simulink model "ACC_simple_model"  (R2018a)
settings: Solver=FixedStepAuto  StartTime=0.0  StopTime=100  RelTol=1e-3
InitFcn:
  | m       = 1800;     % Total mass of vehicle                          (kg)
  | Iz      = 2875;     % Yaw moment of inertia of vehicle               (m*N*s^2)
  | lf      = 1.2;      % Longitudinal distance from c.g. to front tires (m)
  | lr      = 1.6;      % Longitudinal distance from c.g. to rear tires  (m)
  | Cf      = 19000;    % Cornering stiffness of front tires             (N/rad)
  | Cr      = 33000;    % Cornering stiffness of rear tires              (N/rad)
  | tau     = 0.5;      % Longitudinal time constant                     (N/A)
  | 
  | % Initial condition for the ego car
  | v0_ego = 25.6;         % Initial speed of the ego car           (m/s)
  | x0_ego = 0;            % Initial x position of ego car          (m)
  | y0_ego = -757.8;       % Initial y position of ego car          (m)
libraries: simulink x1
settings Model: Creator=CHIZOM WORNU  LastModifiedBy=CHIZOM WORNU
settings OptimizationCC: DefaultParameterBehavior=Inlined  UseDivisionForNetSlopeComputation=on  UseFloatMulNetSlope=on  InlineInvariantSignals=on  PassReuseOutputArgsAs=Individual arguments  ZeroExternalMemoryAtStartup=off  ZeroInternalMemoryAtStartup=off  NoFixptDivByZeroProtection=on  EfficientFloat2IntCast=on  LifeSpan=1  OptimizeBlockOrder=speed  DifferentSizesBufferReuse=on
settings DebuggingCC: ParameterTunabilityLossMsg=error
settings HardwareCC: ProdLongLongMode=on
settings SFSimCC: MATLABDynamicMemAlloc=off
settings RTWCC: SystemTargetFile=ert.tlc  GenCodeOnly=on  PackageName=Accsimple  TemplateMakefile=ert_default_tmf  GenerateReport=on  Toolchain=Microsoft Visual C++ 2017 v15.0 | nmake (64-bit Windows)  IncludeHyperlinkInReport=on  LaunchReport=on  GenerateTraceInfo=on  GenerateTraceReport=on  GenerateTraceReportSl=on  GenerateTraceReportSf=on  GenerateTraceReportEml=on  GenerateCodeMetricsReport=on
settings CodeAppCC: ForceParamTrailComments=on  IgnoreCustomStorageClasses=off  OperatorAnnotations=on  SimulinkDataObjDesc=on  SFDataObjDesc=on  CustomSymbolStrGlobalVar=rt$N$M  CustomSymbolStrType=$N$M  CustomSymbolStrFcn=$N$M$F  CustomSymbolStrMacro=$N$M  InsertBlockDesc=on
settings ERTTargetCC: TargetLangStandard=C99 (ISO)  GenerateSampleERTMain=on  IncludeMdlTerminateFcn=off  CombineSignalStateStructs=on  SupportComplex=off  SupportContinuousTime=on  InlinedParameterPlacement=NonHierarchical  ERTCustomFileTemplate=example_file_process.tlc

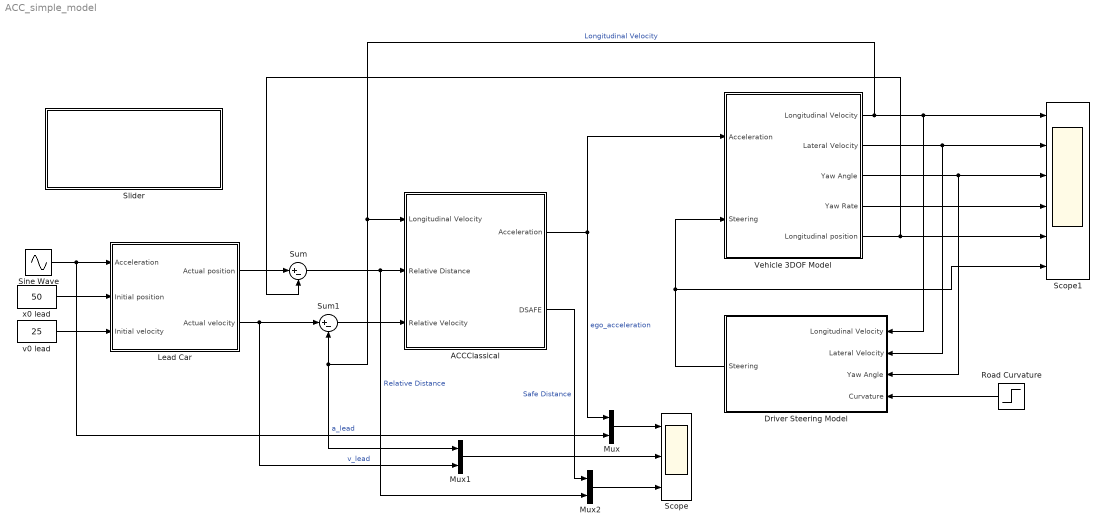
== system ACC_simple_model ==
  "  Vehicle 3DOF Model " : Subsystem
  ACCClassical : Subsystem  TreatAsAtomicUnit=on  VariantControl=controller_type == 1
      settings: RTWFileNameOpts=Use function name
  Driver Steering Model : Subsystem
  Lead Car : Subsystem
  Mux : Mux  Inputs=2
  Mux1 : Mux  Inputs=2
  Mux2 : Mux  Inputs=2
  Road Curvature : Step  Time=50  Before=1/760  After=4/760  SampleTime=0
  Scope : Scope  NumInputPorts=3
  Scope1 : Scope  NumInputPorts=6
  Sine Wave : Sin  Amplitude=0.3188405797101  Frequency=0.2  SampleTime=0.1
  Slider : Subsystem  DialogController=hmiCreateDDGDialog  IsWebBlock=on  mask(MWDashboardBlock){webBlockId=eaa1054b-b6c0-4885-96b6-8836a32feb3e, webBlockType=slider, ShowInLibBrowser=on, ShowInitialText=on, HMISrcModelName=ACC_simple_model}
      mask prompts: webBlockId "WebBlock Id"; webBlockType "WebBlock Type"; HMISrcModelName "Source Model"
      mask help: SimulinkHMI:dialogs:SliderDialogDesc
      mask Help: helpview([docroot '/mapfiles/simulink.map'], 'hmi_slider')
      mask Display:
      | if strcmp(get_param(bdroot(gcb),'BlockDiagramType'), 'library')
      |     image([(matlabroot) '/toolbox/simulink/hmi/icons/Slider.png']);
      | end
  Sum : Sum  Inputs=|+-
  Sum1 : Sum  Inputs=|+-
  v0 lead : Constant  Value=25  SampleTime=0.1
  x0 lead : Constant  Value=50  SampleTime=0.1
  wires:
  Lead Car/2(Actual velocity) -> Sum1/1, Mux1/2  "v_lead"
  Sine Wave/1 -> Mux/2, Lead Car/1(Acceleration)  "a_lead"
  Lead Car/1(Actual position) -> Sum/1
  v0 lead/1 -> Lead Car/3(Initial velocity)
  x0 lead/1 -> Lead Car/2(Initial position)
  ACCClassical/1(Acceleration) -> "  Vehicle 3DOF Model "/1(Acceleration), Mux/1  "ego_acceleration"
  ACCClassical/2("DSAFE ") -> Mux2/1  "Safe Distance"
  Driver Steering Model/1(Steering) -> "  Vehicle 3DOF Model "/2(Steering), Scope1/6
  "  Vehicle 3DOF Model "/1(Longitudinal Velocity) -> Driver Steering Model/1(Longitudinal Velocity), Scope1/1, ACCClassical/1(Longitudinal Velocity), Mux1/1, Sum1/2  "Longitudinal Velocity"
  "  Vehicle 3DOF Model "/2(Lateral Velocity) -> Driver Steering Model/2(Lateral Velocity), Scope1/2
  "  Vehicle 3DOF Model "/3(Yaw Angle) -> Driver Steering Model/3(Yaw Angle), Scope1/3
  "  Vehicle 3DOF Model "/4(Yaw Rate) -> Scope1/4
  "  Vehicle 3DOF Model "/5(Longitudinal position) -> Sum/2, Scope1/5
  Road Curvature/1 -> Driver Steering Model/4(Curvature)
  Mux/1 -> Scope/1
  Mux1/1 -> Scope/2
  Mux2/1 -> Scope/3
  Sum1/1 -> ACCClassical/3(Relative Velocity)
  Sum/1 -> ACCClassical/2(Relative Distance), Mux2/2  "Relative Distance"

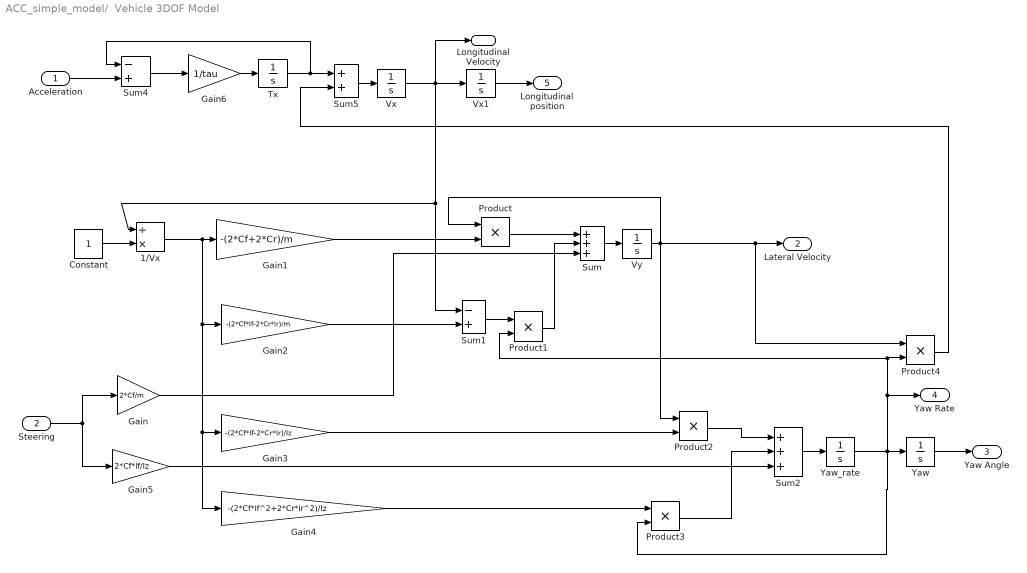
== system ACC_simple_model/  Vehicle 3DOF Model  ==
  Acceleration : Inport
  Steering : Inport  Port=2
  1/Vx : Product  Inputs=/*
  Constant : Constant
  Gain : Gain  Gain=2*Cf/m
  Gain1 : Gain  Gain=-(2*Cf+2*Cr)/m
  Gain2 : Gain  Gain=-(2*Cf*lf-2*Cr*lr)/m
  Gain3 : Gain  Gain=-(2*Cf*lf-2*Cr*lr)/Iz
  Gain4 : Gain  Gain=-(2*Cf*lf^2+2*Cr*lr^2)/Iz
  Gain5 : Gain  Gain=2*Cf*lf/Iz
  Gain6 : Gain  Gain=1/tau
  Product{,1..4} (5 alike) : Product
  Sum : Sum  Inputs=+++
  Sum1 : Sum  Inputs=-+
  Sum2 : Sum  Inputs=+++
  Sum4 : Sum  Inputs=-+
  Sum5 : Sum
  Tx : Integrator
  Vx : Integrator  InitialCondition=v0_ego
  Vx1 : Integrator  InitialCondition=v0_ego
  Vy : Integrator
  Yaw : Integrator
  "Yaw_rate " : Integrator
  Longitudinal Velocity : Outport
  Lateral Velocity : Outport  Port=2
  Yaw Angle : Outport  Port=3
  Yaw Rate : Outport  Port=4
  Longitudinal position : Outport  Port=5
  wires:
  Vx/1 -> 1/Vx/1, Sum1/1, Vx1/1, Longitudinal Velocity/1
  Vy/1 -> Product/1, Product4/1, Lateral Velocity/1, Product2/1
  Yaw/1 -> Yaw Angle/1
  "Yaw_rate "/1 -> Product4/2, Product1/2, Yaw Rate/1, Product3/2, Yaw/1
  Vx1/1 -> Longitudinal position/1
  Product1/1 -> Sum/2
  Sum/1 -> Vy/1
  Product/1 -> Sum/1
  Gain1/1 -> Product/2
  Steering/1 -> Gain/1, Gain5/1
  Gain/1 -> Sum/3
  Sum1/1 -> Product1/1
  Product4/1 -> Sum5/2
  Gain5/1 -> Sum2/3
  Product3/1 -> Sum2/2
  Tx/1 -> Sum5/1, Sum4/1
  Acceleration/1 -> Sum4/2
  Sum4/1 -> Gain6/1
  Product2/1 -> Sum2/1
  1/Vx/1 -> Gain1/1, Gain4/1, Gain3/1, Gain2/1
  Gain3/1 -> Product2/2
  Constant/1 -> 1/Vx/2
  Gain4/1 -> Product3/1
  Gain2/1 -> Sum1/2
  Sum5/1 -> Vx/1
  Sum2/1 -> "Yaw_rate "/1
  Gain6/1 -> Tx/1

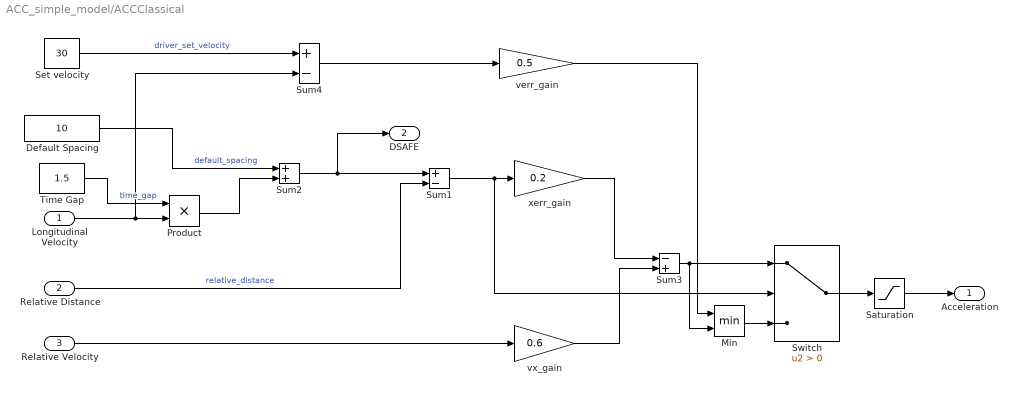
== system ACC_simple_model/ACCClassical ==
  Longitudinal Velocity : Inport
  Relative Distance : Inport  Port=2
  Relative Velocity : Inport  Port=3
  Default Spacing : Constant  Value=10  SampleTime=0.1
  Min : MinMax  Inputs=2
  Product : Product
  Saturation : Saturate  UpperLimit=2  LowerLimit=-3
  Set velocity : Constant  Value=30  SampleTime=0.1
  Sum1 : Sum  Inputs=+-
  Sum2 : Sum
  Sum3 : Sum  Inputs=-+
  Sum4 : Sum  Inputs=+-
  Switch : Switch  Criteria=u2 > Threshold
  Time Gap : Constant  Value=1.5  SampleTime=0.1
  verr_gain : Gain  Gain=0.5
  vx_gain : Gain  Gain=0.6
  xerr_gain : Gain  Gain=0.2
  Acceleration : Outport
  "DSAFE " : Outport  Port=2
  wires:
  Longitudinal Velocity/1 -> Product/2, Sum4/2
  Default Spacing/1 -> Sum2/1  "default_spacing"
  xerr_gain/1 -> Sum3/1
  Sum4/1 -> verr_gain/1
  Min/1 -> Switch/3
  vx_gain/1 -> Sum3/2
  Switch/1 -> Saturation/1
  Relative Velocity/1 -> vx_gain/1
  Time Gap/1 -> Product/1  "time_gap"
  Saturation/1 -> Acceleration/1
  Product/1 -> Sum2/2
  Set velocity/1 -> Sum4/1  "driver_set_velocity"
  Sum3/1 -> Min/2, Switch/1
  Sum1/1 -> Switch/2, xerr_gain/1
  verr_gain/1 -> Min/1
  Relative Distance/1 -> Sum1/2  "relative_distance"
  Sum2/1 -> "DSAFE "/1, Sum1/1

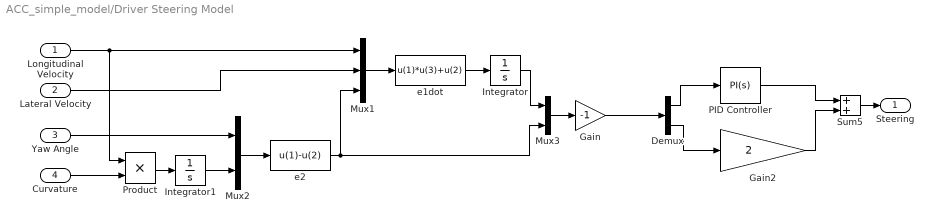
== system ACC_simple_model/Driver Steering Model ==
  Longitudinal Velocity : Inport
  Lateral Velocity : Inport  Port=2
  Yaw Angle : Inport  Port=3
  Curvature : Inport  Port=4
  Demux : Demux  Outputs=2
  Gain : Gain  Gain=-1
  Gain2 : Gain  Gain=2
  Integrator : Integrator
  Integrator1 : Integrator
  Mux1 : Mux  Inputs=3
  Mux2 : Mux  Inputs=2
  Mux3 : Mux  Inputs=2
  PID Controller : simulink/Continuous/PID Controller  Controller=PI  TimeDomain=Continuous-time  SampleTime=-1  IntegratorMethod=Forward Euler  FilterMethod=Forward Euler  Form=Parallel  UseFilter=on  ControllerParametersSource=internal  P=0.2  I=0.1  D=0  N=100  InitialConditionSource=internal  InitialConditionForIntegrator=0  InitialConditionForFilter=0  ExternalReset=none  LimitOutput=off  UpperSaturationLimit=inf  LowerSaturationLimit=-inf  LinearizeAsGain=on  AntiWindupMode=none  Kb=1  TrackingMode=off  Kt=1  PParamMin=[]  PParamMax=[]  IParamMin=[]  IParamMax=[]  DParamMin=[]  DParamMax=[]  NParamMin=[]  NParamMax=[]  KbParamMin=[]  KbParamMax=[]  KtParamMin=[]  KtParamMax=[]  POutMin=[]  POutMax=[]  IOutMin=[]  IOutMax=[]  DOutMin=[]  DOutMax=[]  NOutMin=[]  NOutMax=[]  KbOutMin=[]  KbOutMax=[]  KtOutMin=[]  KtOutMax=[]  IntegratorOutMin=[]  IntegratorOutMax=[]  FilterOutMin=[]  FilterOutMax=[]  SumOutMin=[]  SumOutMax=[]  SumI1OutMin=[]  SumI1OutMax=[]  SumI2OutMin=[]  SumI2OutMax=[]  SumI3OutMin=[]  SumI3OutMax=[]  SumDOutMin=[]  SumDOutMax=[]  SaturationOutMin=[]  SaturationOutMax=[]  IntegratorContinuousStateAttributes=''  IntegratorStateMustResolveToSignalObject=off  IntegratorRTWStateStorageClass=Auto  FilterContinuousStateAttributes=''  FilterStateMustResolveToSignalObject=off  FilterRTWStateStorageClass=Auto  DifferentiatorICPrevScaledInput=0  DifferentiatorOutMin=[]  DifferentiatorOutMax=[]  InitialConditionSetting=State (most efficient)  FilterDiffOutCoefMin=[]  FilterDiffOutCoefMax=[]  SumDenOutMin=[]  SumDenOutMax=[]  SumNumOutMin=[]  SumNumOutMax=[]  ReciprocalOutMin=[]  ReciprocalOutMax=[]  DivideOutMin=[]  DivideOutMax=[]  TunerSelectOption=Transfer Function Based (PID Tuner App)
  Product : Product
  Sum5 : Sum
  e1dot : Fcn  Expr=u(1)*u(3)+u(2)
  e2 : Fcn  Expr=u(1)-u(2)
  Steering : Outport
  wires:
  e1dot/1 -> Integrator/1
  Mux2/1 -> e2/1
  e2/1 -> Mux3/2, Mux1/3
  Mux3/1 -> Gain/1
  Lateral Velocity/1 -> Mux1/2
  Yaw Angle/1 -> Mux2/1
  Mux1/1 -> e1dot/1
  Integrator/1 -> Mux3/1
  Product/1 -> Integrator1/1
  Integrator1/1 -> Mux2/2
  Curvature/1 -> Product/2
  Longitudinal Velocity/1 -> Product/1, Mux1/1
  Gain2/1 -> Sum5/2
  PID Controller/1 -> Sum5/1
  Demux/2 -> Gain2/1
  Sum5/1 -> Steering/1
  Demux/1 -> PID Controller/1
  Gain/1 -> Demux/1

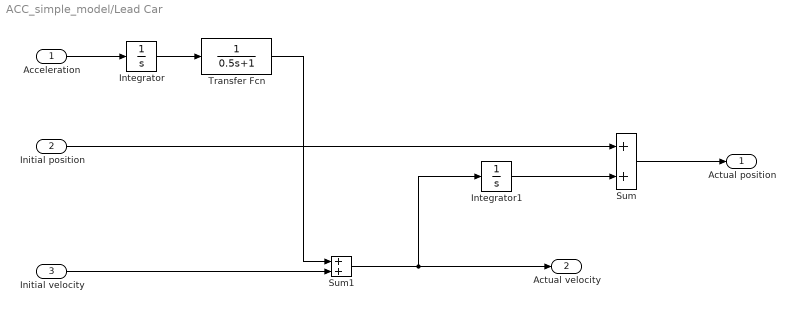
== system ACC_simple_model/Lead Car ==
  Acceleration : Inport
  Initial position : Inport  Port=2
  Initial velocity : Inport  Port=3
  Integrator : Integrator
  Integrator1 : Integrator
  Sum : Sum
  Sum1 : Sum
  Transfer Fcn : TransferFcn  Denominator=[0.5 1]
  Actual position : Outport
  Actual velocity : Outport  Port=2
  wires:
  Transfer Fcn/1 -> Sum1/1
  Initial velocity/1 -> Sum1/2
  Sum/1 -> Actual position/1
  Integrator/1 -> Transfer Fcn/1
  Sum1/1 -> Integrator1/1, Actual velocity/1
  Acceleration/1 -> Integrator/1
  Initial position/1 -> Sum/1
  Integrator1/1 -> Sum/2

== system ACC_simple_model/Slider ==
